simulink model "Factorial_StateFlow"  (R2018a)
settings: Solver=FixedStepDiscrete  StartTime=0.0  StopTime=10.0  RelTol=1e-3
settings Model: Creator=Moataz  LastModifiedBy=Moataz
settings OptimizationCC: DefaultParameterBehavior=Inlined  EnhancedBackFolding=on  PassReuseOutputArgsAs=Individual arguments  OptimizeBlockOrder=speed  DifferentSizesBufferReuse=on  OptimizationCustomize=off
settings DebuggingCC: ParameterTunabilityLossMsg=error
settings SFSimCC: MATLABDynamicMemAlloc=off
settings RTWCC: SystemTargetFile=ert.tlc  GenCodeOnly=on  TemplateMakefile=ert_default_tmf  GenerateReport=on  IncludeHyperlinkInReport=on  LaunchReport=on  GenerateTraceInfo=on  GenerateTraceReport=on  GenerateTraceReportSl=on  GenerateTraceReportSf=on  GenerateTraceReportEml=on
settings CodeAppCC: ForceParamTrailComments=on  IgnoreCustomStorageClasses=off  OperatorAnnotations=on  SimulinkDataObjDesc=on  SFDataObjDesc=on  InsertBlockDesc=on
settings ERTTargetCC: TargetLangStandard=C99 (ISO)  GenerateSampleERTMain=on  InlinedParameterPlacement=NonHierarchical  ERTCustomFileTemplate=example_file_process.tlc

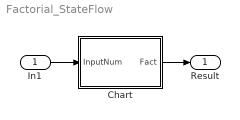
== system Factorial_StateFlow ==
  In1 : Inport  OutDataTypeStr=uint16
  Chart : Stateflow chart  TreatAsAtomicUnit=on
  Result : Outport  OutDataTypeStr=uint16
  wires:
  Chart/1(Fact) -> Result/1
  In1/1 -> Chart/1(InputNum)

== stateflow chart Factorial_StateFlow/Chart ==
  (default) -> (junction 7) : % Factorial_While
      | {Num=InputNum;
      | Fact = uint16(1);}
  (junction 7) -> (junction 9)
  (junction 9) -> (junction 8) [order 1] : [Num>0]
  (junction 8) -> (junction 10) : {Fact*=Num;}
  (junction 10) -> (junction 9) : {Num-= 1;}
  (junction 9) -> (junction 11) [order 2]
  data: InputNum input uint16; Num local uint16 =0; Fact output uint16
